simulink model "dew_sim_2019a"  (R2019a)
settings: Solver=ode15s  StartTime=0.0  StopTime=tsim  RelTol=1e-2
values from neighbouring files (symbols this model uses):
  A_1_low = 0.50    (= 0.5)    [simulation_dew.m]
  A_1_mid = A_1_max - A_1_min    (= 0.79)    [simulation_dew.m]
  A_1_min = 0.21    [simulation_dew.m]
  A_1_upp = 1    [simulation_dew.m]
  Estrategia = 1    [simulation_dew.m]
  G_1_low = 0.30    (= 0.3)    [simulation_dew.m]
  G_1_mid = G_1_max - G_1_min    (= 0.4)    [simulation_dew.m]
  G_1_min = 0.2    [simulation_dew.m]
  G_1_upp = 0.50    (= 0.5)    [simulation_dew.m]
  Kec = 0.0050866    [dew_simulink.m]    (also in dewasme_unified.m = k(3); simulation_dew.m)
  Kio = 5.5526    [dew_simulink.m]    (also in dewasme_unified.m = 4.7323; simulation_dew.m)
  Ks = 0.020908    [dew_simulink.m]    (also in dewasme_unified.m = 0.1414; simulation_dew.m)
  mu_set = 0.11    [simulation_dew.m]
  N_1_low = 0    [simulation_dew.m]
  N_1_max = 300    [simulation_dew.m]
  N_1_min = 300    [simulation_dew.m]
  N_1_upp = 0.30    (= 0.3)    [simulation_dew.m]
  PI_Kd = 0    [simulation_dew.m]
  PI_Kd_2 = 0    [simulation_dew.m]
  PI_Ki = 1163.22932064265    (= 1163.22932064)    [simulation_dew.m]
  PI_Ki_2 = 0.06    [simulation_dew.m]
  PI_Kp = 1.87082881181595    (= 1.87082881182)    [simulation_dew.m]
  PI_Kp_2 = 13.0    (= 13)    [simulation_dew.m]
  qOmax = 0.23447    [dew_simulink.m]    (also in dewasme_unified.m = k(5); simulation_dew.m)
  qSmax = 8.0728    [dew_simulink.m]    (also in dewasme_unified.m = k(1); simulation_dew.m)
  Sfeed = 450    [simulation_dew.m]
  spO2 = 0.3*O2s    (= 0.00238555038055)    [simulation_dew.m]
  Ts = 1/60    (= 0.0166666666667)    [simulation_dew.m]
  u_1_low = 0    [simulation_dew.m]
  u_1_upp = 1    [simulation_dew.m]
  Vin = 0.3    [simulation_dew.m]
  Xin = 4.13    [simulation_dew.m]
  Yeo = 0.87877    [dew_simulink.m]    (also in dewasme_unified.m = 1.998; simulation_dew.m)
  Yex = 0.32087    [dew_simulink.m]    (also in dewasme_unified.m = k(4); simulation_dew.m)
  Yosof = u(16)    [dew_simulink.m]    (also in dewasme_unified.m = 0.0001; simulation_dew.m = 0.00011)
  Yse = u(10)    [dew_simulink.m]    (also in dewasme_unified.m = 0.9634; simulation_dew.m = 1.0303)
  Yso = 0.18711    [dew_simulink.m]    (also in dewasme_unified.m = 0.3438; simulation_dew.m)
  Ysofx = 0.3179    [dew_simulink.m]    (also in dewasme_unified.m = 0.3294; simulation_dew.m)
  Ysoxx = 0.30544    [dew_simulink.m]    (also in dewasme_unified.m = k(2); simulation_dew.m)
undefined symbols (not defined in the file or in its folder): magnitude
libraries: simulink x2
settings Model: OrderedModelArguments=off  Creator=dnavalos  LastModifiedBy=Tomás
settings DebuggingCC: SFMachineParentedDataDiag=error

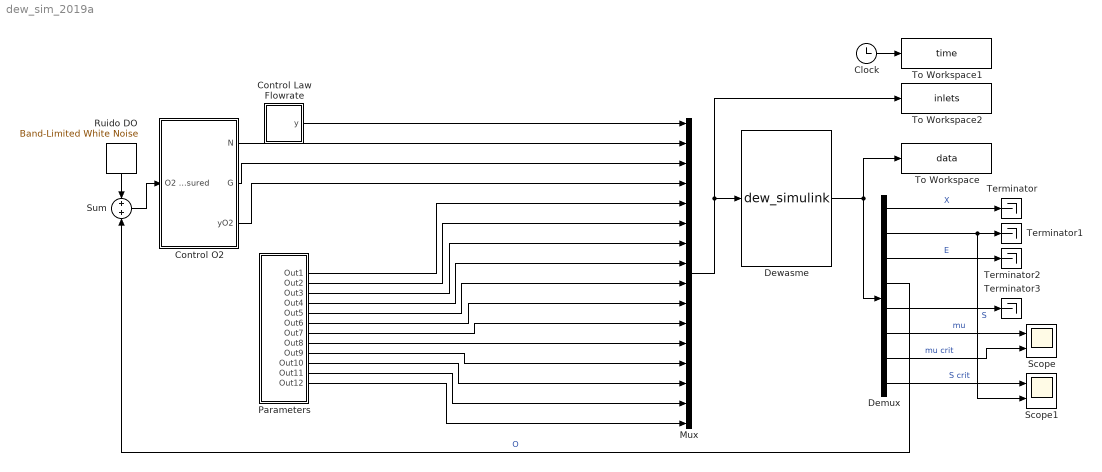
== system dew_sim_2019a ==
  Clock : Clock
  Control Law Flowrate : Subsystem
  Control O2 : Subsystem
  Demux : Demux  Outputs=8
  Dewasme : S-Function  FunctionName=dew_simulink  SFunctionDeploymentMode=off  EnableBusSupport=off
      mask Display: image('reactor.jpg'); % Use "Edit Image" on toolstrip to change.
  Mux : Mux  Inputs=16
  Parameters : Subsystem
  Ruido DO : simulink/Sources/Band-Limited White Noise  Cov=sigma_DO  Ts=Ts  seed=[23341]
  Scope : Scope  NumInputPorts=2
  Scope1 : Scope  NumInputPorts=2
  Sum : Sum
  Terminator{,1..3} (4 alike) : Terminator
  To Workspace : ToWorkspace  VariableName=data  SampleTime=-1
  To Workspace1 : ToWorkspace  VariableName=time  SampleTime=-1
  To Workspace2 : ToWorkspace  VariableName=inlets  SampleTime=-1
  wires:
  Dewasme/1 -> To Workspace/1, Demux/1
  Clock/1 -> To Workspace1/1
  Control Law Flowrate/1(y) -> Mux/1
  Mux/1 -> To Workspace2/1, Dewasme/1
  Control O2/1(N) -> Mux/2
  Control O2/2(G) -> Mux/3
  Control O2/3(yO2) -> Mux/4
  Demux/4 -> Sum/2  "O"
  Sum/1 -> Control O2/1(O2 measured)
  Ruido DO/1 -> Sum/1
  Demux/5 -> Terminator3/1
  Demux/3 -> Terminator2/1  "E"
  Demux/2 -> Scope1/2, Terminator1/1  "S"
  Demux/1 -> Terminator/1  "X"
  Parameters/1(Out1) -> Mux/5
  Parameters/2(Out2) -> Mux/6
  Parameters/3(Out3) -> Mux/7
  Parameters/4(Out4) -> Mux/8
  Parameters/5(Out5) -> Mux/9
  Parameters/6(Out6) -> Mux/10
  Parameters/7(Out7) -> Mux/11
  Parameters/8(Out8) -> Mux/12
  Parameters/9(Out9) -> Mux/13
  Parameters/10(Out10) -> Mux/14
  Parameters/11(Out11) -> Mux/15
  Parameters/12(Out12) -> Mux/16
  Demux/6 -> Scope/1  "mu"
  Demux/7 -> Scope/2  "mu crit"
  Demux/8 -> Scope1/1  "S crit"

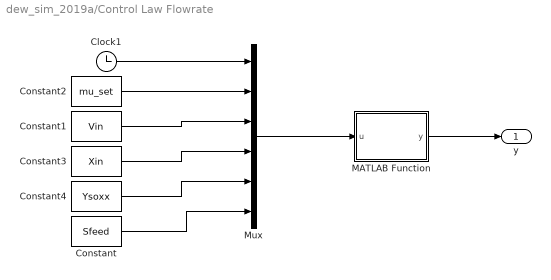
== system dew_sim_2019a/Control Law Flowrate ==
  Clock1 : Clock
  Constant : Constant  Value=Sfeed
  Constant1 : Constant  Value=Vin
  Constant2 : Constant  Value=mu_set
  Constant3 : Constant  Value=Xin
  Constant4 : Constant  Value=Ysoxx
  MATLAB Function : MATLAB Function  TreatAsAtomicUnit=on
  Mux : Mux  Inputs=6
  y : Outport
  wires:
  Constant/1 -> Mux/6
  Constant3/1 -> Mux/4
  Clock1/1 -> Mux/1
  Constant2/1 -> Mux/2
  Constant1/1 -> Mux/3
  Constant4/1 -> Mux/5
  Mux/1 -> MATLAB Function/1(u)
  MATLAB Function/1(y) -> y/1

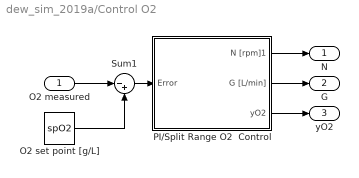
== system dew_sim_2019a/Control O2 ==
  O2 measured : Inport
  O2 set point [g/L] : Constant  Value=spO2
  PI/Split Range O2  Control : Subsystem
  Sum1 : Sum  Inputs=|-+
  N : Outport  VectorParamsAs1DForOutWhenUnconnected=off
  G : Outport  Port=2  VectorParamsAs1DForOutWhenUnconnected=off
  yO2 : Outport  Port=3  VectorParamsAs1DForOutWhenUnconnected=off
  wires:
  PI/Split Range O2  Control/1(N [rpm]1) -> N/1
  PI/Split Range O2  Control/2(G [L/min]) -> G/1
  O2 measured/1 -> Sum1/1
  O2 set point [g/L]/1 -> Sum1/2
  PI/Split Range O2  Control/3("yO2 ") -> yO2/1
  Sum1/1 -> PI/Split Range O2  Control/1(Error)

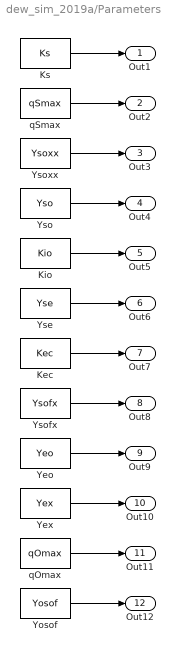
== system dew_sim_2019a/Parameters ==
  Kec : Constant  Value=Kec
  Kio : Constant  Value=Kio
  Ks : Constant  Value=Ks
  Yeo : Constant  Value=Yeo
  Yex : Constant  Value=Yex
  Yosof : Constant  Value=Yosof
  Yse : Constant  Value=Yse
  Yso : Constant  Value=Yso
  Ysofx : Constant  Value=Ysofx
  Ysoxx : Constant  Value=Ysoxx
  qOmax : Constant  Value=qOmax
  qSmax : Constant  Value=qSmax
  Out1 : Outport
  Out2 : Outport  Port=2
  Out3 : Outport  Port=3
  Out4 : Outport  Port=4
  Out5 : Outport  Port=5
  Out6 : Outport  Port=6
  Out7 : Outport  Port=7
  Out8 : Outport  Port=8
  Out9 : Outport  Port=9
  Out10 : Outport  Port=10
  Out11 : Outport  Port=11
  Out12 : Outport  Port=12
  wires:
  Ks/1 -> Out1/1
  qSmax/1 -> Out2/1
  Ysoxx/1 -> Out3/1
  Yso/1 -> Out4/1
  Kio/1 -> Out5/1
  Yse/1 -> Out6/1
  Kec/1 -> Out7/1
  Ysofx/1 -> Out8/1
  Yeo/1 -> Out9/1
  Yex/1 -> Out10/1
  qOmax/1 -> Out11/1
  Yosof/1 -> Out12/1

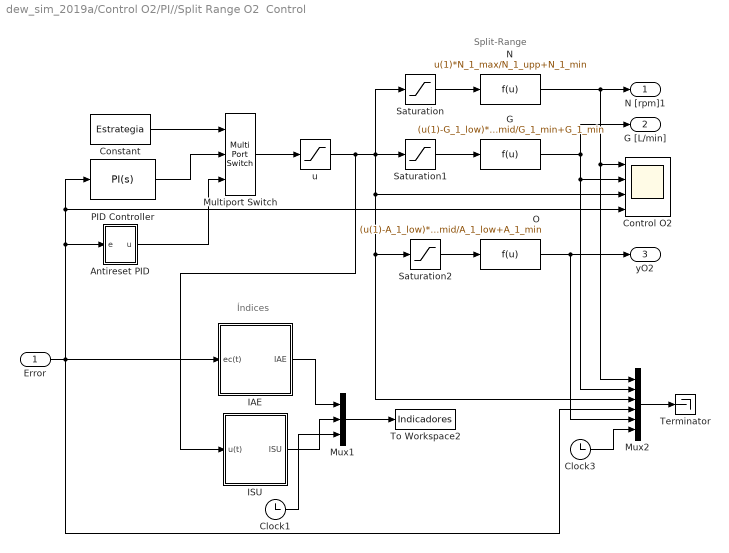
== system dew_sim_2019a/Control O2/PI//Split Range O2  Control ==
  note: Índices
  note: Split-Range
  Error : Inport
  Antireset PID : Subsystem  mask(Antireset PID){G=PI_Kp_2, ti=PI_Ki_2, td=PI_Kd_2, a=0.5, U=1, L=0}
      mask prompts: G "Controller Gain"; ti "Integral Time Constant"; td "Derivative Time Constant"; a "Alpha"; U "Saturation Upper Limit"; L "Saturation Lower Limit"
      mask help: Enter expression for Controller Gain, Integral Time Constant, Derivative Time Constant, Alpha Constant, Saturation Upper Constant, and Saturation Lower Constant terms.
  Clock1 : Clock
  Clock3 : Clock
  Constant : Constant  Value=Estrategia
  Control O2 : Scope  NumInputPorts=4
  G : Fcn  Expr=(u(1)-G_1_low)*G_1_mid/G_1_min+G_1_min
  IAE : Subsystem
  ISU : Subsystem
  Multiport Switch : MultiPortSwitch  Inputs=2
  Mux1 : Mux  Inputs=3
  Mux2 : Mux  Inputs=6
  N : Fcn  Expr=u(1)*N_1_max/N_1_upp+N_1_min
  O : Fcn  Expr=(u(1)-A_1_low)*A_1_mid/A_1_low+A_1_min
  PID Controller : simulink/Continuous/PID Controller  Controller=PI  Form=Parallel  TimeDomain=Continuous-time  SampleTime=-1  IntegratorMethod=Forward Euler  ControllerParametersSource=internal  P=PI_Kp  I=PI_Ki  D=PI_Kd  UseFilter=on  N=479.898765366224  TunerSelectOption=Transfer Function Based (PID Tuner App)  InitialConditionSource=internal  InitialConditionForIntegrator=-48.255  InitialConditionForFilter=0  DifferentiatorICPrevScaledInput=0  ExternalReset=none  TrackingMode=off  Kt=1  LimitOutput=on  UpperSaturationLimit=1  LowerSaturationLimit=0  LinearizeAsGain=off  AntiWindupMode=back-calculation  Kb=1  POutMin=[]  POutMax=[]  IOutMin=[]  IOutMax=[]  DOutMin=[]  DOutMax=[]  NOutMin=[]  NOutMax=[]  SumOutMin=[]  SumOutMax=[]  SaturationOutMin=[]  SaturationOutMax=[]  PParamMin=[]  PParamMax=[]  IParamMin=[]  IParamMax=[]  DParamMin=[]  DParamMax=[]  NParamMin=[]  NParamMax=[]  KbParamMin=[]  KbParamMax=[]  KtParamMin=[]  KtParamMax=[]  KbOutMin=[]  KbOutMax=[]  KtOutMin=[]  KtOutMax=[]  IntegratorOutMin=[]  IntegratorOutMax=[]  FilterOutMin=[]  FilterOutMax=[]  SumI1OutMin=[]  SumI1OutMax=[]  SumI2OutMin=[]  SumI2OutMax=[]  SumI3OutMin=[]  SumI3OutMax=[]  SumI4OutMin=[]  SumI4OutMax=[]  SumDOutMin=[]  SumDOutMax=[]  DifferentiatorOutMin=[]  DifferentiatorOutMax=[]  FilterDiffOutCoefMin=[]  FilterDiffOutCoefMax=[]  ReciprocalOutMin=[]  ReciprocalOutMax=[]  SumDenOutMin=[]  SumDenOutMax=[]  SumNumOutMin=[]  SumNumOutMax=[]  DivideOutMin=[]  DivideOutMax=[]  IntegratorContinuousStateAttributes=''  IntegratorStateMustResolveToSignalObject=off  IntegratorRTWStateStorageClass=Auto  FilterContinuousStateAttributes=''  FilterStateMustResolveToSignalObject=off  FilterRTWStateStorageClass=Auto  ParallelPVariant=InternalParameters  IdealPVariant=Disabled  IVariant=InternalParameters  DVariant=Disabled  IntegratorVariant=Continuous  SatVariant=Enabled  AWVariant=BackCalculation  PCopyVariant=Disabled  TRVariant=Disabled  FdbkBlocksVariant=Forward  IdealPFdbkVariant=Disabled  SatFdbkVariant=Disabled  DerivativeFilterVariant=Disabled  NVariant=Disabled  NCopyVariant=Disabled_SignalSpec  FilterICVariant=Disabled  IntegratorICVariant=InternalICs  ExternalResetVariant=Disabled  TRSumVariant=Passthrough  SumFdbkVariant=Disabled  SumVariant=Sum_PI
  Saturation : Saturate  UpperLimit=N_1_upp  LowerLimit=N_1_low
  Saturation1 : Saturate  UpperLimit=G_1_upp  LowerLimit=G_1_low
  Saturation2 : Saturate  UpperLimit=A_1_upp  LowerLimit=A_1_low
  Terminator : Terminator
  To Workspace2 : ToWorkspace  VariableName=Indicadores  SampleTime=-1
  u : Saturate  UpperLimit=u_1_upp  LowerLimit=u_1_low
  N [rpm]1 : Outport  VectorParamsAs1DForOutWhenUnconnected=off
  G [L/min] : Outport  Port=2  VectorParamsAs1DForOutWhenUnconnected=off
  "yO2 " : Outport  Port=3  VectorParamsAs1DForOutWhenUnconnected=off
  wires:
  Saturation2/1 -> O/1
  Constant/1 -> Multiport Switch/1
  Clock3/1 -> Mux2/6
  N/1 -> N [rpm]1/1, Mux2/1, Control O2/1
  Multiport Switch/1 -> u/1
  ISU/1(ISU) -> Mux1/2
  IAE/1(IAE) -> Mux1/1
  Clock1/1 -> Mux1/3
  Mux1/1 -> To Workspace2/1
  Mux2/1 -> Terminator/1
  PID Controller/1 -> Multiport Switch/2
  Saturation1/1 -> G/1
  Saturation/1 -> N/1
  O/1 -> Mux2/5, "yO2 "/1
  Antireset PID/1(u) -> Multiport Switch/3
  u/1 -> ISU/1(u(t)), Saturation/1, Saturation1/1, Mux2/3, Saturation2/1, Control O2/3
  G/1 -> G [L/min]/1, Mux2/2, Control O2/2
  Error/1 -> PID Controller/1, Control O2/4, Antireset PID/1(e), Mux2/4, IAE/1(ec(t))

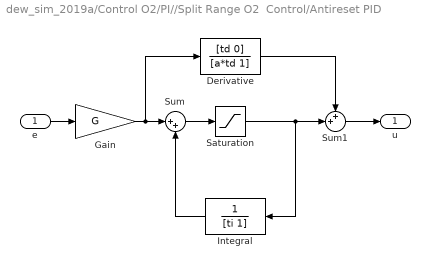
== system dew_sim_2019a/Control O2/PI//Split Range O2  Control/Antireset PID ==
  e : Inport
  Derivative : TransferFcn  Numerator=[td 0]  Denominator=[a*td 1]
  Gain : Gain  Gain=G  SaturateOnIntegerOverflow=on  OutDataTypeStr=Inherit: Same as input  ParamDataTypeStr=Inherit: Same as input
  Integral : TransferFcn  Denominator=[ti 1]
  Saturation : Saturate  UpperLimit=U  LowerLimit=L
  Sum : Sum  Inputs=|++  InputSameDT=on  SaturateOnIntegerOverflow=on  OutDataTypeStr=Inherit: Same as first input
  Sum1 : Sum  Inputs=++|  InputSameDT=on  SaturateOnIntegerOverflow=on  OutDataTypeStr=Inherit: Same as first input
  u : Outport  VectorParamsAs1DForOutWhenUnconnected=off
  wires:
  Derivative/1 -> Sum1/1
  Sum1/1 -> u/1
  Saturation/1 -> Integral/1, Sum1/2
  e/1 -> Gain/1
  Integral/1 -> Sum/2
  Sum/1 -> Saturation/1
  Gain/1 -> Derivative/1, Sum/1

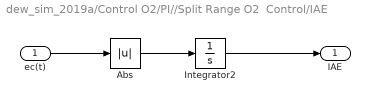
== system dew_sim_2019a/Control O2/PI//Split Range O2  Control/IAE ==
  ec(t) : Inport
  Abs : Abs
  Integrator2 : Integrator
  IAE : Outport  VectorParamsAs1DForOutWhenUnconnected=off
  wires:
  Abs/1 -> Integrator2/1
  ec(t)/1 -> Abs/1
  Integrator2/1 -> IAE/1

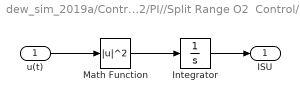
== system dew_sim_2019a/Control O2/PI//Split Range O2  Control/ISU ==
  u(t) : Inport
  Integrator : Integrator
  Math Function : Math  Operator=magnitude^2  SaturateOnIntegerOverflow=on
  ISU : Outport  VectorParamsAs1DForOutWhenUnconnected=off
  wires:
  Integrator/1 -> ISU/1
  u(t)/1 -> Math Function/1
  Math Function/1 -> Integrator/1

== matlab function dew_sim_2019a/Control Law Flowrate/MATLAB Function ==
  data: u input; y output
function y = fcn(u)
t = u(1);
muset= u(2); Vin = u(3); Xin = u(4);
Ysoxx = u(5); Sin = u(6);

F0      = muset*(Xin*Vin)/(Ysoxx*Sin);
F       = F0*exp(muset*t);

y = F;
end
